simulink model "FEDNNSimulacion"  (R2022b)
settings: Solver=VariableStepAuto  StartTime=0.0  StopTime=30  FixedStep=0.0001  RelTol=1e-3
values from neighbouring files (symbols this model uses):
  A = A + size * eye(size)    [FEDNN_viga_index.m]    (also in IniciadorOchoEstados.m = [zeros(r,r),eye(r); IniciadorParametros.m = [zeros(nq,nq),eye(nq); beam2.m = [zeros(nq,nq),eye(nq))
  B = [zeros(r,m) ... (first row only)    [IniciadorOchoEstados.m]    (also in IniciadorParametros.m = [zeros(nq,m); beam2.m = [zeros(nq,m))
  f = 4    [IniciadorOchoEstados.m]    (also in IniciadorParametros.m = 19)
  k1 = 1    [IniciadorOchoEstados.m]    (also in IniciadorParametros.m = 2.2802)
  k2 = 1/2    (= 0.5)    [IniciadorOchoEstados.m]    (also in IniciadorParametros.m = 2.7468)
  ne = 20    [IniciadorParametros.m]    (also in beam2.m = 21)
  nq = dof*(nn-nbc)    [IniciadorParametros.m]    (also in beam2.m)
  P = I    [FEDNN_viga_index.m]    (also in UnaPquesifunciona.mat = [65.2176366949 7.33136484028 -7.82447895775 3.52933243114 5.)
  W1_0 = rand(E,E)    [IniciadorOchoEstados.m]    (also in IniciadorParametros.m = rand(n,n))
  W2_0 = rand(E,E)    [IniciadorOchoEstados.m]    (also in IniciadorParametros.m = rand(n,n))
settings Model: Creator=raul  LastModifiedBy=raul

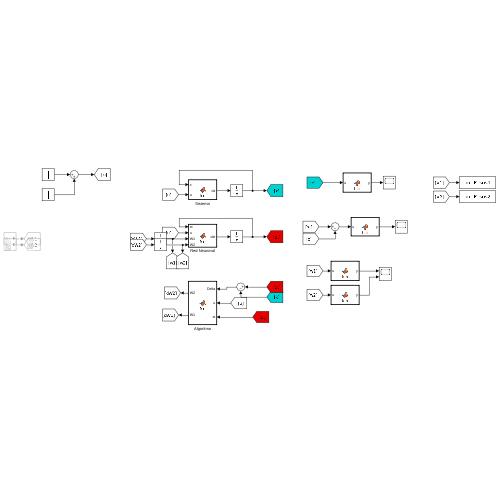
[thumbnail: Simulink's stored preview of the top-level diagram]
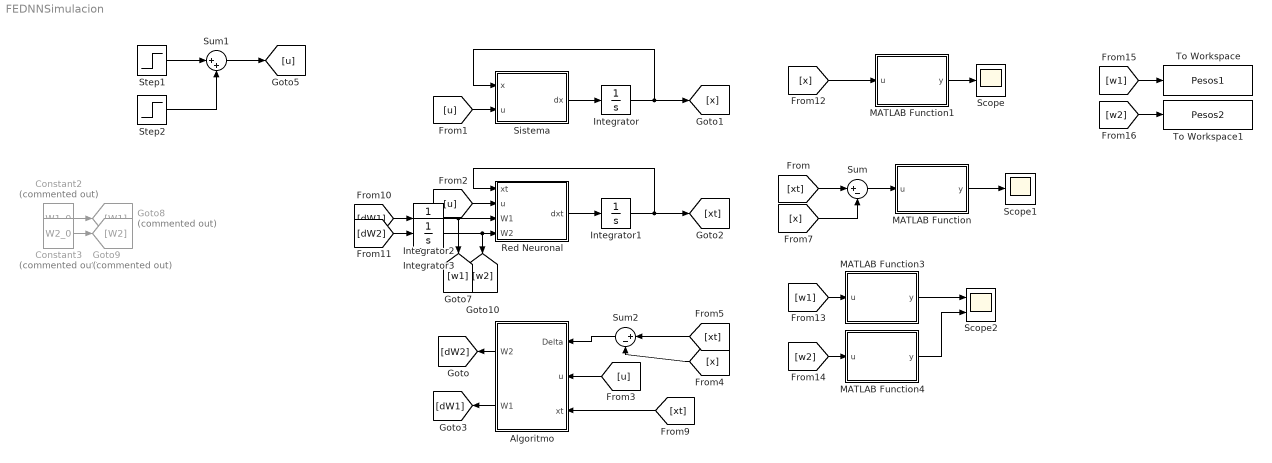
== system FEDNNSimulacion ==
  Algoritmo : MATLAB Function  TreatAsAtomicUnit=on
  Constant2 : Constant  Commented=on  Value=W1_0
  Constant3 : Constant  Commented=on  Value=W2_0
  Goto8 : Goto  Commented=on  GotoTag=W1
  Goto9 : Goto  Commented=on  GotoTag=W2
  Integrator : Integrator  InitialCondition=zeros(2*ne,ne)
  Integrator1 : Integrator  InitialCondition=zeros(2*nq,20)
  Integrator2 : Integrator  InitialCondition=W1_0
  Integrator3 : Integrator  InitialCondition=W2_0
  MATLAB Function : MATLAB Function  TreatAsAtomicUnit=on
  MATLAB Function1 : MATLAB Function  TreatAsAtomicUnit=on
  MATLAB Function3 : MATLAB Function  TreatAsAtomicUnit=on
  MATLAB Function4 : MATLAB Function  TreatAsAtomicUnit=on
  Red Neuronal : MATLAB Function  TreatAsAtomicUnit=on
  Scope : Scope
  Scope1 : Scope
  Scope2 : Scope  NumInputPorts=2
  Sistema : MATLAB Function  TreatAsAtomicUnit=on
  Step1 : Step  SampleTime=0
  Step2 : Step  Time=1.1  After=-1  SampleTime=0
  Sum : Sum  Inputs=|+-
  Sum1 : Sum  Inputs=|++
  Sum2 : Sum  Inputs=|+-
  To Workspace : ToWorkspace  VariableName=Pesos1  SampleTime=-1
  To Workspace1 : ToWorkspace  VariableName=Pesos2  SampleTime=-1
  wires:
  Step2/1 -> Sum1/2
  Step1/1 -> Sum1/1
  Sistema/1(dx) -> Integrator/1
  Integrator/1 -> [x], Sistema/1(x)
  [xt] -> Sum/1
  [x] -> Sum/2
  Red Neuronal/1(dxt) -> Integrator1/1
  Integrator1/1 -> [xt], Red Neuronal/1(xt)
  Sum1/1 -> [u]
  [u] -> Sistema/2(u)
  [u] -> Red Neuronal/2(u)
  [u] -> Algoritmo/2(u)
  Sum2/1 -> Algoritmo/1(Delta)
  [x] -> Sum2/2
  [xt] -> Sum2/1
  Algoritmo/1(W2) -> [dW2]
  Algoritmo/2(W1) -> [dW1]
  [xt] -> Algoritmo/3(xt)
  Constant2/1 -> Goto8/1
  Constant3/1 -> Goto9/1
  Sum/1 -> MATLAB Function/1(u)
  MATLAB Function/1(y) -> Scope1/1
  MATLAB Function1/1(y) -> Scope/1
  [x] -> MATLAB Function1/1(u)
  Integrator3/1 -> [w2], Red Neuronal/4(W2)
  Integrator2/1 -> [w1], Red Neuronal/3(W1)
  [dW2] -> Integrator3/1
  [dW1] -> Integrator2/1
  [w1] -> MATLAB Function3/1(u)
  MATLAB Function3/1(y) -> Scope2/1
  [w2] -> MATLAB Function4/1(u)
  MATLAB Function4/1(y) -> Scope2/2
  [w2] -> To Workspace1/1
  [w1] -> To Workspace/1

== matlab function FEDNNSimulacion/Algoritmo ==
  data: W2 output; Delta input; P parameter; u input; W1 output; k1 parameter; k2 parameter; xt input
function [W2,W1] = fcn(Delta,P,u, k1, k2,xt)


W1=-k1*P*Delta*sigmoid(1,xt)';
W2=-k2*P*Delta*sigmoid(1,xt)'*u;


% function [du, dW, dV] = DNN(u, us, W1, V1, h)
% 	Delta   = u - us;
% 	sigma   = sigmoid(1,V1*u);
% 	D_sigma = diag(sigma.*(1-sigma));
% 	%
% 	dW      = h*(-K1NN*PNN*Delta*sigma' + K1NN*PNN*Delta*u'*(V1-V0NN)'*D_sigma);
% 	dV		= h*(-K2NN*D_sigma'*W1'*PNN*Delta*u' - lNN/2*K2NN*LambdaNN*(V1-V0NN)*(u*u'));
% 	du		= h*(ANN*u + W1*sigma);
% end


function s = sigmoid(b,x)
   s = 1./(1+exp(-b*x)); 
end

end

== matlab function FEDNNSimulacion/Red Neuronal ==
  data: xt input; u input; dxt output; W1 input; A parameter; W2 input
function dxt = fcn(xt, u, W1, A, W2)

dxt = A*xt+W1*sigmoid(1,xt)+W2*sigmoid(1,xt)*u;


function s = sigmoid(b,x)
   s = 1./(1+exp(-b*x)); 
end

end

== matlab function FEDNNSimulacion/Sistema ==
  data: x input; u input; dx output; A parameter; B parameter; f parameter
function dx = fcn(x,u,A, B, f)%add Bw,w

dx = A*x+B*u;

%dx = A*x+B(:,f)*u+Bw*w;

== matlab function FEDNNSimulacion/MATLAB Function ==
  data: u input; y output
function y = fcn(u)

y = u(:,20);

== matlab function FEDNNSimulacion/MATLAB Function1 ==
  data: u input; y output; f parameter
function y = fcn(u,f)

y = u(:,f);

== matlab function FEDNNSimulacion/MATLAB Function3 ==
  data: u input; y output; f parameter
function y = fcn(u,f)

y = u(:,f);

== matlab function FEDNNSimulacion/MATLAB Function4 ==
  data: u input; y output; f parameter
function y = fcn(u,f)

y = u(:,f);
